simulink model "AirSys_Lib"  (R2016b)
settings: configuration reference "CodeGenConfigSet" (kept outside this file)
settings Model: Creator=GaberXu  LastModifiedBy=GaberXu
settings ConfigSetRef: SourceLocation=Base Workspace

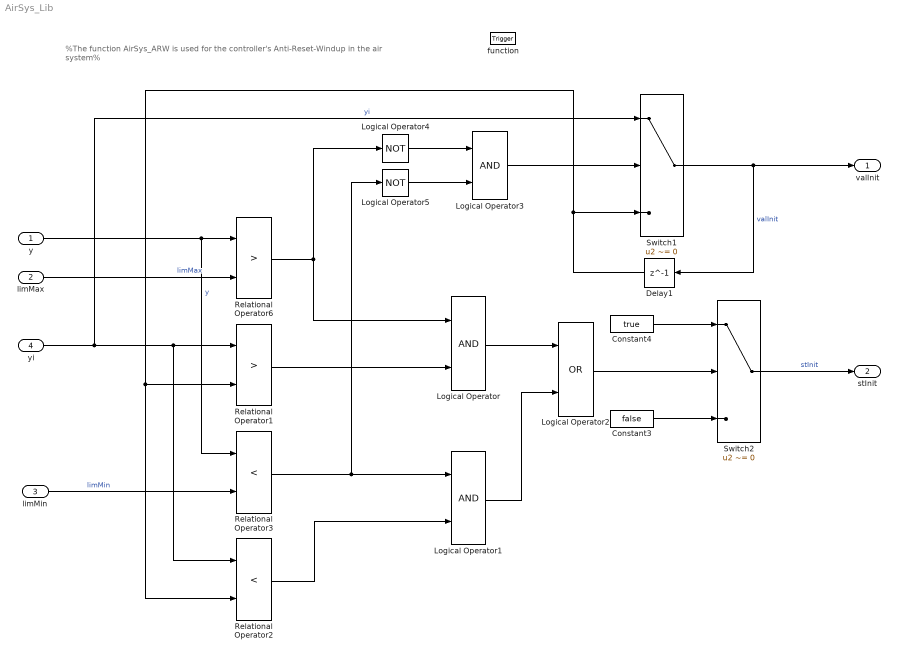
== system AirSys_Lib ==
  note: %The function AirSys_ARW is used for the controller's Anti-Reset-Windup in the air system%
  y : Inport  Description=Controller correcting variable  OutMin=-32768  OutMax=32767  OutDataTypeStr=State_int16
  limMax : Inport  Description=Maximum limitation of the controller correcting variable  Port=2  OutMin=-32768  OutMax=32767  OutDataTypeStr=State_int16
  limMin : Inport  Description=Minimum limitation of the controller correcting variable  Port=3  OutMin=-32768  OutMax=32767  OutDataTypeStr=State_int16
  yi : Inport  Description=I-component of the controller correcting variable  Port=4  OutMin=-32768  OutMax=32767  OutDataTypeStr=State_int16
  function : TriggerPort  TriggerType=function-call  VariantControl=Variant
  Constant3 : Constant  RequirementInfo={'other' 'APP_requirements.doc' '@Simulink_requirement_item_25' 'true' '手动开关' '' } %GIDa_ccc40e8c_f875_4ea9_b16c_df72cac2f315  Value=false  OutDataTypeStr=boolean
  Constant4 : Constant  RequirementInfo={'other' 'APP_requirements.doc' '@Simulink_requirement_item_25' 'true' '手动开关' '' } %GIDa_587c3a58_10cc_42f3_9e55_69c7f436f0a3  Value=true  OutDataTypeStr=boolean
  Delay1 : Delay  DelayLength=1
  Logical Operator : Logic  OutDataTypeStr=boolean
  Logical Operator1 : Logic  OutDataTypeStr=boolean
  Logical Operator2 : Logic  Operator=OR  OutDataTypeStr=boolean
  Logical Operator3 : Logic  OutDataTypeStr=boolean
  Logical Operator4 : Logic  Operator=NOT  AllPortsSameDT=off  OutDataTypeStr=boolean
  Logical Operator5 : Logic  Operator=NOT  AllPortsSameDT=off  OutDataTypeStr=boolean
  Relational Operator1 : RelationalOperator  Operator=>  OutDataTypeStr=boolean  RndMeth=Simplest  InputSameDT=on
  Relational Operator2 : RelationalOperator  Operator=<  OutDataTypeStr=boolean  RndMeth=Simplest  InputSameDT=on
  Relational Operator3 : RelationalOperator  Operator=<  OutDataTypeStr=boolean  RndMeth=Simplest  InputSameDT=on
  Relational Operator6 : RelationalOperator  Operator=>  OutDataTypeStr=boolean  RndMeth=Simplest  InputSameDT=on
  Switch1 : Switch  Criteria=u2 ~= 0  InputSameDT=on
      settings: AttributesFormatString=InputSameDT=%<InputSameDT>
  Switch2 : Switch  Criteria=u2 ~= 0  InputSameDT=on
      settings: AttributesFormatString=InputSameDT=%<InputSameDT>
  valInit : Outport  Description=Initialization value for active ARW  OutMin=-32768  OutMax=32767  OutDataTypeStr=State_int16
  stInit : Outport  Description=State ARW (1 = active, 0 = inactive)  Port=2  OutMin=0  OutMax=1  OutDataTypeStr=boolean
  wires:
  Constant3/1 -> Switch2/3
  Switch1/1 -> valInit/1, Delay1/1  "valInit"
  Logical Operator2/1 -> Switch2/2
  Relational Operator1/1 -> Logical Operator/2
  Constant4/1 -> Switch2/1
  Switch2/1 -> stInit/1  "stInit"
  Logical Operator3/1 -> Switch1/2
  limMin/1 -> Relational Operator3/2  "limMin"
  Logical Operator4/1 -> Logical Operator3/1
  y/1 -> Relational Operator3/1, Relational Operator6/1  "y"
  limMax/1 -> Relational Operator6/2  "limMax"
  Logical Operator5/1 -> Logical Operator3/2
  Logical Operator/1 -> Logical Operator2/1
  Logical Operator1/1 -> Logical Operator2/2
  Relational Operator3/1 -> Logical Operator1/1, Logical Operator5/1
  Delay1/1 -> Switch1/3, Relational Operator1/2, Relational Operator2/2
  yi/1 -> Relational Operator2/1, Relational Operator1/1, Switch1/1  "yi"
  Relational Operator2/1 -> Logical Operator1/2
  Relational Operator6/1 -> Logical Operator4/1, Logical Operator/1
